simulink model "myfirstsimulinkfilec_control101"  (R2023b)
settings: Solver=VariableStepAuto  StartTime=0.0  StopTime=endtime  RelTol=1e-3
undefined symbols (not defined in the file): d, Kp, n
settings Model: Creator=Anthony  LastModifiedBy=Anthony Rossiter
settings DataIOCC: SaveFormat=Array

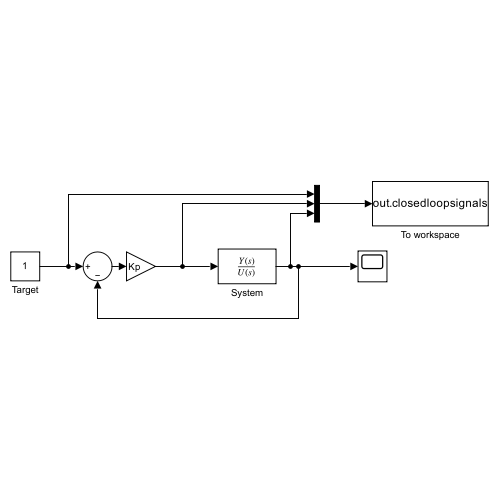
[thumbnail: Simulink's stored preview of the top-level diagram]
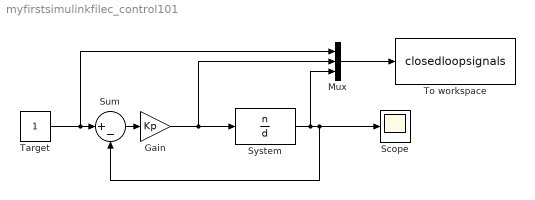
== system myfirstsimulinkfilec_control101 ==
  Gain : Gain  Gain=Kp
  Mux : Mux  Inputs=3
  Scope : Scope
  Sum : Sum  Inputs=|+-
  System : TransferFcn  Numerator=n  Denominator=d
  Target : Constant
  To workspace : ToWorkspace  VariableName=closedloopsignals  SaveFormat=Timeseries  SampleTime=-1
  wires:
  Gain/1 -> Mux/2, System/1
  System/1 -> Mux/3, Scope/1, Sum/2
  Mux/1 -> To workspace/1
  Target/1 -> Mux/1, Sum/1
  Sum/1 -> Gain/1
